simulink model "PI1"  (R2022a)
settings: Solver=VariableStepAuto  StartTime=0.0  StopTime=0.3  RelTol=1e-3
values from neighbouring files (symbols this model uses):
  c1 = k * 0.75e-9    (= 1.7175e-09)    [hinf_design.m]    (also in system_parameters.mat = -16.5; system_parameters_3d.mat = -16.5)
  fs = 30000    [system_parameters.mat]    (also in system_parameters_3d.mat = 20000)
libraries: simulink x1
settings Model: Creator=doamarar  LastModifiedBy=doamarar

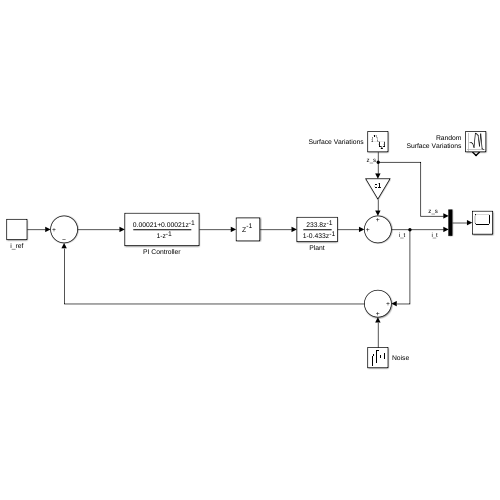
[thumbnail: Simulink's stored preview of the top-level diagram]
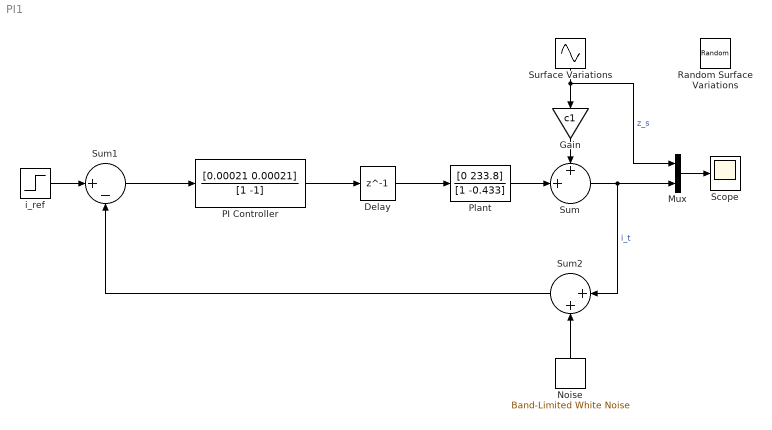
== system PI1 ==
  Delay : Delay  DelayLength=1  SampleTime=1/fs
  Gain : Gain  Gain=c1
  Mux : Mux  Inputs=2
  Noise : simulink/Sources/Band-Limited White Noise  Cov=[0.0000000000000000000000000001]  Ts=1/fs  seed=[23341]
  PI Controller : DiscreteFilter  Numerator=[0.00021 0.00021]  Denominator=[1 -1]  SampleTime=1/fs
  Plant : DiscreteFilter  Numerator=[0 233.8]  Denominator=[1 -0.433]  FilterStructure=Direct form I  SampleTime=1/fs
  Random Surface Variations : RandomNumber  Variance=2*10^-25  SampleTime=1/fs
  Scope : Scope
  Sum : Sum  Inputs=++|
  Sum1 : Sum  Inputs=|+-
  Sum2 : Sum  Inputs=|++
  Surface Variations : Sin  Amplitude=2.5*10^-11  Frequency=600  SampleTime=1/fs
  i_ref : Step  Time=0  After=0.25*10^-9  SampleTime=1/fs
  wires:
  Delay/1 -> Plant/1
  Plant/1 -> Sum/2
  Sum/1 -> Mux/2, Sum2/1  "i_t"
  i_ref/1 -> Sum1/1
  Sum1/1 -> PI Controller/1
  Noise/1 -> Sum2/2
  Surface Variations/1 -> Mux/1, Gain/1  "z_s"
  Sum2/1 -> Sum1/2
  PI Controller/1 -> Delay/1
  Gain/1 -> Sum/1
  Mux/1 -> Scope/1
